simulink model "Pumpmotorrotordynamics"  (R2025b)
settings: Solver=ode45  StartTime=0.0  StopTime=1000  FixedStep=1  RelTol=1e-3
undefined symbols (not defined in the file): alpha_Q, eta_p, g, H_pump_m, J_total, K_H, N_motor_rpm, N_ref, Q_design, Q_pump, rho, T_motor_Nm
settings Model: Creator=admin  LastModifiedBy=admin

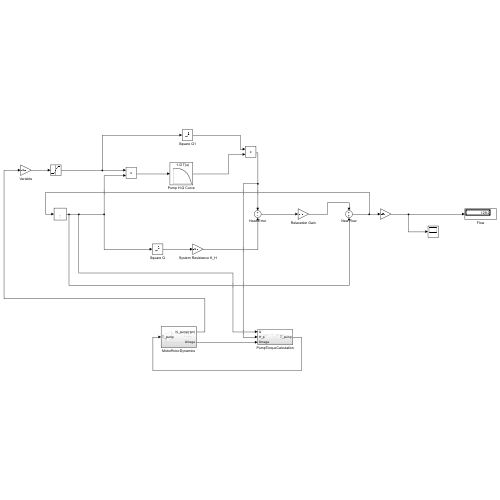
[thumbnail: Simulink's stored preview of the top-level diagram]
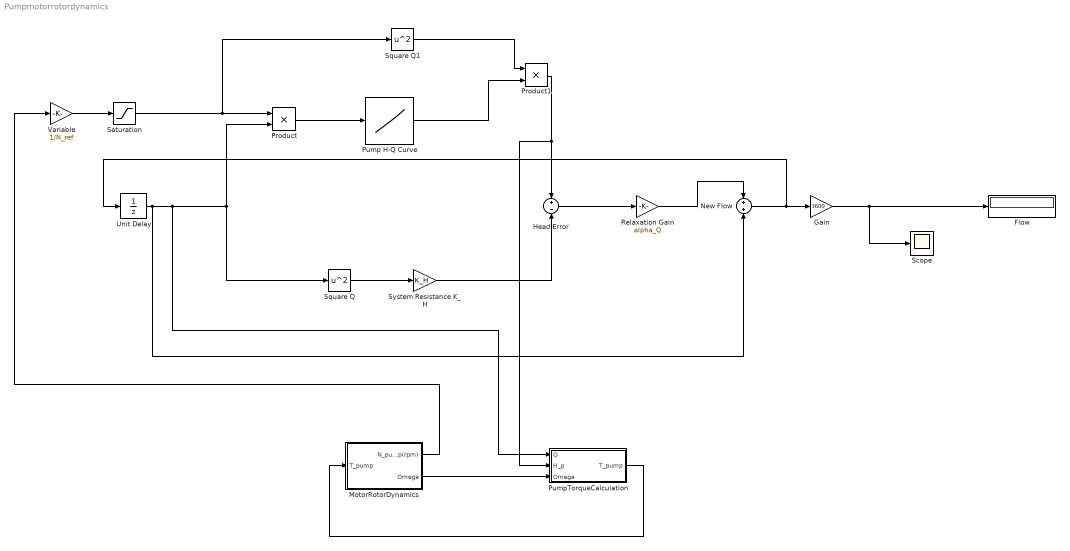
== system Pumpmotorrotordynamics ==
  Flow : Display
  Gain : Gain  Gain=3600
  Head Error : Sum  Inputs=+-
  MotorRotorDynamics : Subsystem
  New Flow : Sum
  Product : Product
  Product1 : Product
  Pump H-Q Curve : Lookup_n-D  NumberOfTableDimensions=1  BreakpointsForDimension1=Q_pump  Table=H_pump_m  InternalRulePriority=Speed  RndMeth=Simplest
  PumpTorqueCalculation : Subsystem
  Relaxation Gain : Gain  Gain=alpha_Q
  Saturation : Saturate  UpperLimit=1.2  LowerLimit=0.01
  Scope : Scope
      settings: ActiveDisplayYMinimum=43.172229326381718  ActiveDisplayYMaximum=150.793190621606
  Square Q : Math  Operator=square
  Square Q1 : Math  Operator=square
  System Resistance K_H : Gain  Gain=K_H
  Unit Delay : UnitDelay  InitialCondition=Q_design  HasFrameUpgradeWarning=on
  Variable : Gain  Gain=1/N_ref
  wires:
  Pump H-Q Curve/1 -> Product1/2
  Square Q/1 -> System Resistance K_H/1
  System Resistance K_H/1 -> Head Error/2
  Unit Delay/1 -> New Flow/2, PumpTorqueCalculation/1(Q), Product/2, Square Q/1
  Head Error/1 -> Relaxation Gain/1
  Relaxation Gain/1 -> New Flow/1
  New Flow/1 -> Unit Delay/1, Gain/1
  Gain/1 -> Scope/1, Flow/1
  Product/1 -> Pump H-Q Curve/1
  Saturation/1 -> Square Q1/1, Product/1
  Square Q1/1 -> Product1/1
  Product1/1 -> PumpTorqueCalculation/2(H_p), Head Error/1
  MotorRotorDynamics/1(N_pump(rpm)) -> Variable/1
  MotorRotorDynamics/2(Omega) -> PumpTorqueCalculation/3(Omega)
  PumpTorqueCalculation/1(T_pump) -> MotorRotorDynamics/1(T_pump)
  Variable/1 -> Saturation/1

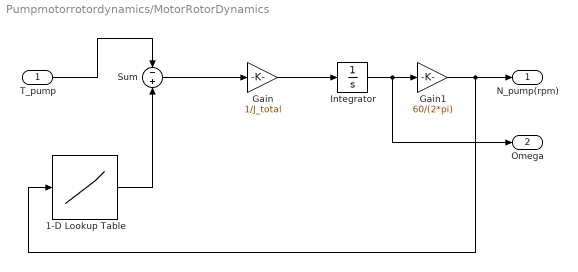
== system Pumpmotorrotordynamics/MotorRotorDynamics ==
  T_pump : Inport
  1-D Lookup Table : Lookup_n-D  NumberOfTableDimensions=1  BreakpointsForDimension1=N_motor_rpm  Table=T_motor_Nm  InternalRulePriority=Speed  RndMeth=Simplest
  Gain : Gain  Gain=1/J_total
  Gain1 : Gain  Gain=60/(2*pi)
  Integrator : Integrator
  Sum : Sum  Inputs=-+
  N_pump(rpm) : Outport
  Omega : Outport  Port=2
  wires:
  T_pump/1 -> Sum/1
  Sum/1 -> Gain/1
  Gain/1 -> Integrator/1
  Integrator/1 -> Omega/1, Gain1/1
  Gain1/1 -> 1-D Lookup Table/1, N_pump(rpm)/1
  1-D Lookup Table/1 -> Sum/2

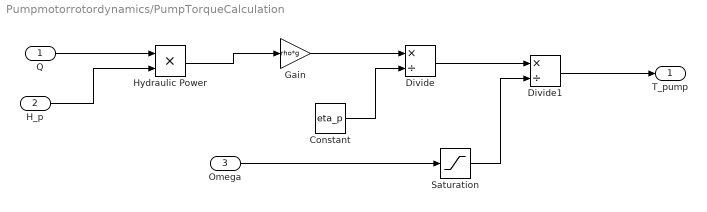
== system Pumpmotorrotordynamics/PumpTorqueCalculation ==
  Q : Inport
  H_p : Inport  Port=2
  Omega : Inport  Port=3
  Constant : Constant  Value=eta_p
  Divide : Product  Inputs=*/
  Divide1 : Product  Inputs=*/
  Gain : Gain  Gain=rho*g
  Hydraulic Power : Product
  Saturation : Saturate  UpperLimit=inf  LowerLimit=1
  T_pump : Outport
  wires:
  Hydraulic Power/1 -> Gain/1
  Gain/1 -> Divide/1
  Divide/1 -> Divide1/1
  Saturation/1 -> Divide1/2
  Q/1 -> Hydraulic Power/1
  H_p/1 -> Hydraulic Power/2
  Omega/1 -> Saturation/1
  Constant/1 -> Divide/2
  Divide1/1 -> T_pump/1
